simulink model "liti4_701"  (Simulink 5.0)
settings: Solver=ode45  SolverMode=SingleTasking  StartTime=0.0  StopTime=3  FixedStep=0.1  RelTol=1e-3
libraries: cstblocks x2
settings Model: LastModifiedBy=Administrator

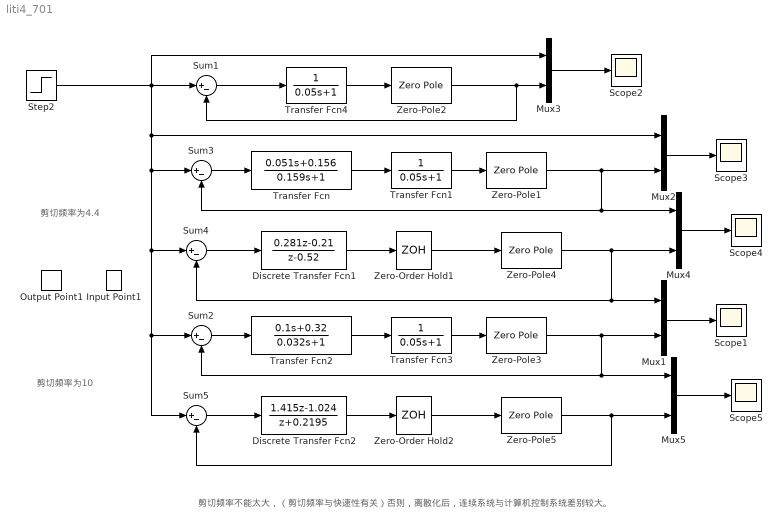
== system liti4_701 ==
  note: 剪切频率不能太大，（剪切频率与快速性有关）否则，离散化后，连续系统与计算机控制系统差别较大。
  note: 剪切频率为10
  note: 剪切频率为4.4
  Discrete Transfer Fcn1 : DiscreteTransferFcn  Numerator=[0.281 -0.21]  Denominator=[1 -0.52]  SampleTime=0.1
  Discrete Transfer Fcn2 : DiscreteTransferFcn  Numerator=[1.415 -1.024]  Denominator=[1 0.2195]  SampleTime=0.1
  Input Point1 : cstblocks/Input Point
  Mux{1..5} (5 alike) : Mux  Inputs=2
  Output Point1 : cstblocks/Output Point
  Scope{1..5} (5 alike) : Scope
      Scope1 settings: YMin=-3.5  YMax=1  MaxDataPoints=500000
      Scope2 settings: YMin=-3.5  YMax=1  MaxDataPoints=500000
      Scope3 settings: YMin=-3.5  YMax=1  SaveName=ScopeData2  MaxDataPoints=500000
      Scope4 settings: YMin=-3.5  YMax=1  SaveName=yyy  DataFormat=Array  MaxDataPoints=500000
      Scope5 settings: YMin=-3.5  YMax=1  SaveName=yyy1  DataFormat=Array  MaxDataPoints=500000
  Step2 : Step  Time=0  SampleTime=0
  Sum{1..5} (5 alike) : Sum  Inputs=|+-  SaturateOnIntegerOverflow=on
  Transfer Fcn : TransferFcn  Numerator=[0.051 0.156]  Denominator=[0.159 1]
  Transfer Fcn1 : TransferFcn  Denominator=[0.05 1]
  Transfer Fcn2 : TransferFcn  Numerator=[0.1 0.32]  Denominator=[0.032 1]
  Transfer Fcn3 : TransferFcn  Denominator=[0.05 1]
  Transfer Fcn4 : TransferFcn  Denominator=[0.05 1]
  Zero-Order Hold1 : ZeroOrderHold  SampleTime=0.1
  Zero-Order Hold2 : ZeroOrderHold  SampleTime=0.1
  Zero-Pole{1..5} (5 alike) : ZeroPole  Zeros=[]  Poles=[0 -4]  Gain=[120]
  wires:
  Step2/1 -> Mux3/1, Sum1/1, Mux2/1, Sum3/1, Sum4/1, Sum5/1, Sum2/1
  Mux2/1 -> Scope3/1
  Zero-Pole1/1 -> Mux2/2, Sum3/2, Mux4/1
  Transfer Fcn/1 -> Transfer Fcn1/1
  Transfer Fcn1/1 -> Zero-Pole1/1
  Mux3/1 -> Scope2/1
  Zero-Pole2/1 -> Mux3/2, Sum1/2
  Sum1/1 -> Transfer Fcn4/1
  Sum3/1 -> Transfer Fcn/1
  Mux4/1 -> Scope4/1
  Zero-Pole4/1 -> Mux4/2, Sum4/2, Mux1/1
  Discrete Transfer Fcn1/1 -> Zero-Order Hold1/1
  Sum4/1 -> Discrete Transfer Fcn1/1
  Zero-Order Hold1/1 -> Zero-Pole4/1
  Mux1/1 -> Scope1/1
  Zero-Pole3/1 -> Mux5/1, Sum2/2, Mux1/2
  Transfer Fcn2/1 -> Transfer Fcn3/1
  Transfer Fcn3/1 -> Zero-Pole3/1
  Sum2/1 -> Transfer Fcn2/1
  Mux5/1 -> Scope5/1
  Zero-Pole5/1 -> Sum5/2, Mux5/2
  Discrete Transfer Fcn2/1 -> Zero-Order Hold2/1
  Sum5/1 -> Discrete Transfer Fcn2/1
  Zero-Order Hold2/1 -> Zero-Pole5/1
  Transfer Fcn4/1 -> Zero-Pole2/1
